simulink model "SimHydraulics_Cylinder_Pump_3"  (R2014a)
settings: Solver=ode45  StartTime=0.0  StopTime=10.0  RelTol=1e-3
libraries: sh_lib x4, fl_lib x3, nesl_utility x2
Description:
  | Copyright 2014 The MathWorks, Inc.
settings Model: Creator=smiller  LastModifiedBy=smiller
settings DataIOCC: SignalLoggingSaveFormat=ModelDataLogs
settings OptimizationCC: ExpressionDepthLimit=2147483647  InitFltsAndDblsToZero=on
settings DebuggingCC: SaveWithParameterizedLinksMsg=none  UnderspecifiedInitializationDetection=Classic  FcnCallInpInsideContextMsg=UseLocalSettings  StateNameClashWarn=warning
settings GRTTargetCC: TargetFcnLib=ansi_tfl_tmw.mat  CombineOutputUpdateFcns=off  GRTInterface=on

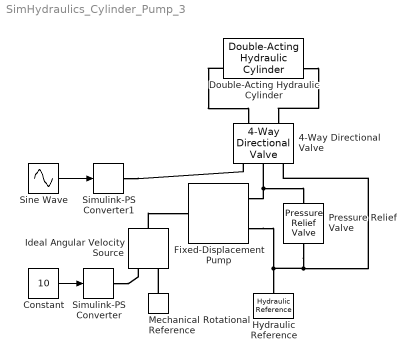
== system SimHydraulics_Cylinder_Pump_3 ==
  4-Way Directional Valve : sh_lib/Valves/Directional Valves/4-Way Directional Valve  Tag=Factory Generic  mdl_type=1  area_max=1e-05 m^2  opening_max=0.005 m  opening_tab="[  -0.002 0 0.005 0.015 ] m"  area_tab="[  1e-12 4e-12 1e-05 1.02e-05 ] m^2"  pressure_tab="[  -5e+06 -2e+06 2e+06 5e+06 ] Pa"  flow_rate_tab="[  -1e-12 -6e-14 6e+12 1e+11 ; -8e-08 -4e-08 4e+06 8e+06 ; -0.0025 -0.00103 0.001 0.0024 ; -0.00258 -0.001032 0.00106 0.00247 ; ] m^3/s"  interp_method=1  extrap_method=1  C_d=0.7  x_0_P_A=0 m  x_0_P_B=0 m  x_0_A_T=0 m  x_0_B_T=0 m  Re_cr=12  A_leak=1e-9 m^2
  Constant : Constant  Value=10
  Double-Acting Hydraulic Cylinder : sh_lib/Hydraulic Cylinders/Double-Acting Hydraulic Cylinder  area_A=5e-04 m^2  area_B=5e-04 m^2  stroke=0.2 m  init_pos=0.1 m  dead_vol_A=1e-04 m^3  dead_vol_B=1e-04 m^3  init_pressure_A=0 Pa  init_pressure_B=0 Pa  k_sh=1.4  stiff=1e+06 N/m  D=150 N/(m/s)  or=1  or_sign=1
  Fixed-Displacement Pump : sh_lib/Pumps and Motors/Fixed-Displacement Pump  D=5e-06 m^3/rad  efficiency_vol=0.92  efficiency_tot=0.8  pr_nominal=1e+07 Pa  w_nominal=188 rad/s  visc_nominal=18 cSt  dens_nominal=900 kg/m^3  k_leak=1e-11 m^3/s/Pa  efficiency_mech=0.7
  Hydraulic Reference : fl_lib/Hydraulic/Hydraulic Elements/Hydraulic Reference  Tag=Factory Generic
  Ideal Angular Velocity Source : fl_lib/Mechanical/Mechanical Sources/Ideal Angular Velocity Source
  Mechanical Rotational Reference : fl_lib/Mechanical/Rotational Elements/Mechanical Rotational Reference
  Pressure Relief Valve : sh_lib/Valves/Pressure Control Valves/Pressure Relief Valve  area_max=1e-04 m^2  pres_set=1e5 Pa  reg_range=1e4 Pa  C_d=0.7  Re_cr=12  A_leak=1e-12 m^2  gain=1 m^2/Pa  pr_max=55e5 Pa
  Simulink-PS Converter : nesl_utility/Simulink-PS Converter  PhysicalDomain=network_engine_domain  SubClassName=ps_input  LeftPortType=input  RightPortType=output  PseudoPeriodic=off  Frequencies=[]  NoiseDistribution=none  NoiseParameters=[]  Unit=rad/s  AffineConversion=off  InputFiltering=off  SimscapeFilterOrder=1  InputFilterTimeConstant=.001  UdotUserProvided=0
  Simulink-PS Converter1 : nesl_utility/Simulink-PS Converter  PhysicalDomain=network_engine_domain  SubClassName=ps_input  LeftPortType=input  RightPortType=output  PseudoPeriodic=off  Frequencies=[]  NoiseDistribution=none  NoiseParameters=[]  Unit=m  AffineConversion=off  InputFiltering=off  SimscapeFilterOrder=1  InputFilterTimeConstant=.001  UdotUserProvided=0
  Sine Wave : Sin  Amplitude=0.005  SampleTime=0
  wires:
  Sine Wave/1 -> Simulink-PS Converter1/1
  Constant/1 -> Simulink-PS Converter/1
  connections:
  4-Way Directional Valve/RConn3 -- Pressure Relief Valve/RConn1 -- Fixed-Displacement Pump/RConn2 -- Hydraulic Reference/LConn1
  Fixed-Displacement Pump/RConn1 -- 4-Way Directional Valve/RConn2 -- Pressure Relief Valve/LConn1
  Double-Acting Hydraulic Cylinder/LConn2 -- 4-Way Directional Valve/LConn1
  Simulink-PS Converter1/RConn1 -- 4-Way Directional Valve/RConn1
  Ideal Angular Velocity Source/LConn1 -- Fixed-Displacement Pump/LConn1
  Double-Acting Hydraulic Cylinder/RConn2 -- 4-Way Directional Valve/LConn2
  Simulink-PS Converter/RConn1 -- Ideal Angular Velocity Source/RConn1
  Mechanical Rotational Reference/LConn1 -- Ideal Angular Velocity Source/RConn2
